simulink model "sim"  (R2024b)
settings: Solver=VariableStepAuto  StartTime=0.0  StopTime=10.0  RelTol=1e-3
settings Model: Creator=Ishak  LastModifiedBy=Ishak

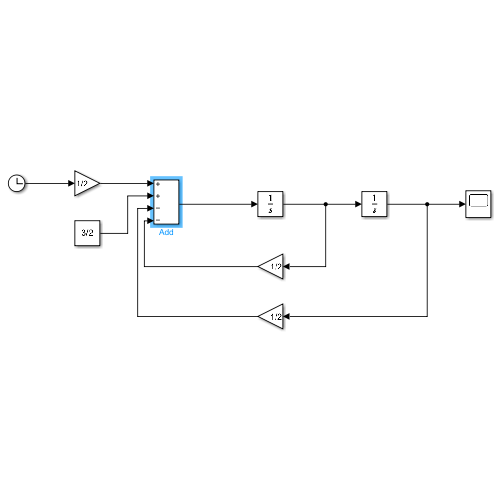
[thumbnail: Simulink's stored preview of the top-level diagram]
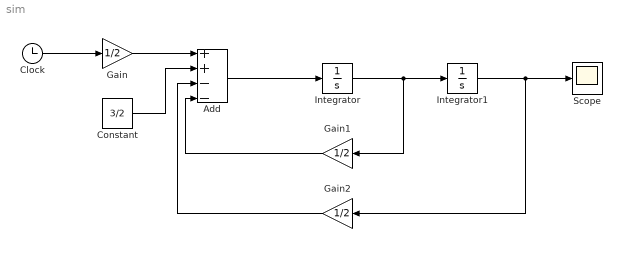
== system sim ==
  Add : Sum  Inputs=++--
  Clock : Clock
  Constant : Constant  Value=3/2
  Gain : Gain  Gain=1/2
  Gain1 : Gain  Gain=1/2
  Gain2 : Gain  Gain=1/2
  Integrator : Integrator  InitialCondition=1
  Integrator1 : Integrator  InitialCondition=2
  Scope : Scope
  wires:
  Add/1 -> Integrator/1
  Integrator/1 -> Gain1/1, Integrator1/1
  Gain/1 -> Add/1
  Clock/1 -> Gain/1
  Constant/1 -> Add/2
  Gain1/1 -> Add/4
  Integrator1/1 -> Gain2/1, Scope/1
  Gain2/1 -> Add/3
